simulink model "KIT_pr_UDR"  (R2023a)
settings: Solver=VariableStepAuto  StartTime=0.0  StopTime=inf  RelTol=1e-3
values from neighbouring files (symbols this model uses):
  Cx_alpha = [-0.0016 -0.0039 0.0346]    [KIT_UDR.mat]
  Cy_alpha = [-0.0006 0.0037 0.1555 0.2133]    [KIT_UDR.mat]
  InertiaTensor = [0.41697  0  0; 0  0.27367  0; 0  0  0.15697]    [KIT_UDR.mat]
  Mass = 3    [KIT_UDR.mat]
  mz_alpha = [-2e-05 0.0001 -0.0017 0.0042]    [KIT_UDR.mat]
  square = 0.228    [KIT_UDR.mat]
undefined symbols (not defined in the file or in its folder): deg, e0_0, e1_0, e2_0, e3_0, PitchAngleToTorque, rad, RollAngleToTorque, s, YawAngleToTorque
libraries: aerolibconvert2 x9, dsppolyfun x3, aerolibanimutils x3, sharedutil x2, etargetslib x1, aerolibutil x1, dspnetwork x1
settings Model: Creator=Sony  LastModifiedBy=sasha
settings SolverCC: AlgebraicLoopSolver=TrustRegion  DecoupledContinuousIntegration=on  MinimalZcImpactIntegration=on
settings DebuggingCC: ReadBeforeWriteMsg=DisableAll  WriteAfterWriteMsg=DisableAll  WriteAfterReadMsg=DisableAll  MultiTaskDSMMsg=none  UnconnectedInputMsg=warning  UnconnectedOutputMsg=warning  UnconnectedLineMsg=warning  ArithmeticOperatorsInVariantConditions=warning
settings ModelReferenceCC: UpdateModelReferenceTargets=IfOutOfDate  EnableRefExpFcnMdlSchedulingChecks=on
settings SFSimCC: SFSimEcho=off  CustomCodeUndefinedFunction=UseInterfaceOnly
settings RTWCC: DLArmComputeVersion=19.05
settings CodeAppCC: StateflowObjectComments=on

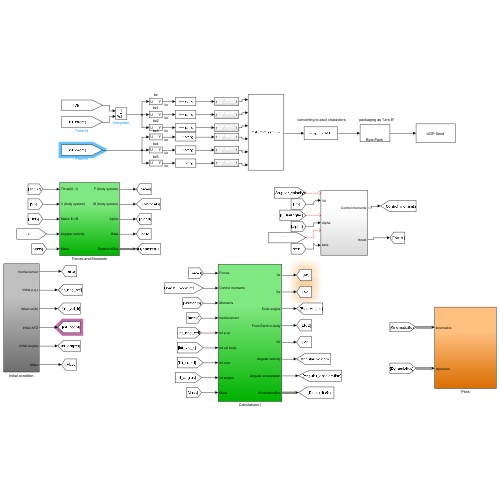
[thumbnail: Simulink's stored preview of the top-level diagram]
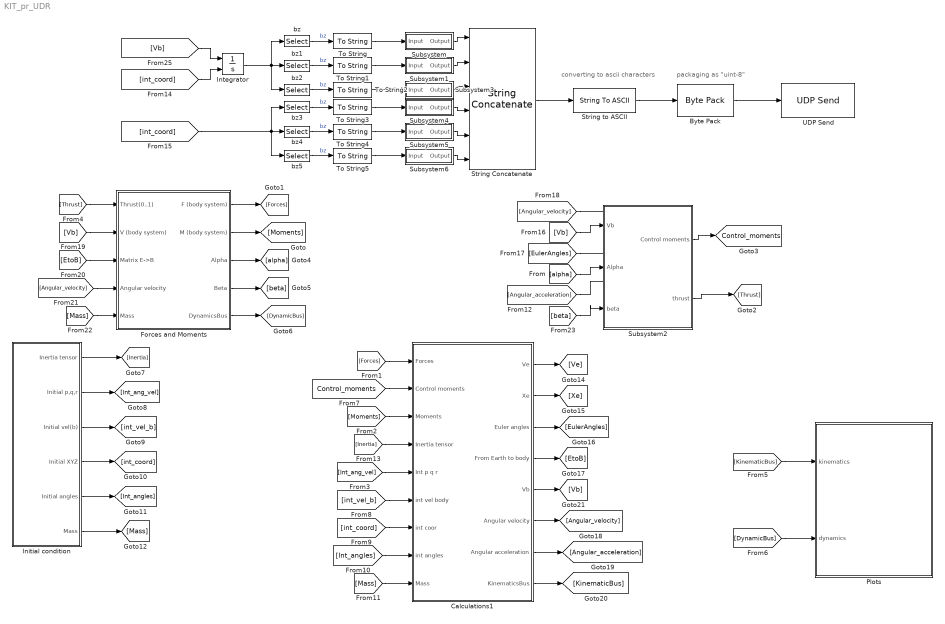
== system KIT_pr_UDR ==
  note: packaging as "uint-8"
  note: converting to ascii characters
  Byte Pack : etargetslib/Byte Pack  datatypes={'uint8'}  byteAlign=1
  Calculations1 : Subsystem
  Forces and Moments : Subsystem
  Initial condition : Subsystem
  Integrator : Integrator  InitialConditionSource=external
  Plots : Subsystem
  String Concatenate : StringConcatenate  Inputs=6
  String to ASCII : StringToASCII  OutputVectorSize=64
  Subsystem : Subsystem
  Subsystem1 : Subsystem
  Subsystem2 : Subsystem
  Subsystem3 : Subsystem
  Subsystem4 : Subsystem
  Subsystem5 : Subsystem
  Subsystem6 : Subsystem
  To String{,1..5} (6 alike) : ToString
  UDP Send : dspnetwork/UDP Send  remoteURL='127.0.0.1'  remotePort=1234  localURL='0.0.0.0'  localPortSource=Automatically determine  localPort=-1  sendBufferSize=8192  sampletime=-1  blockPlatform=[]  separateLengthPort=0
      settings: LibrarySourceBlock=dspsnks4/UDP Send
  bz : Selector  InputPortWidth=3  IndexOptions=Index vector (dialog)  Indices=1  OutputSizes=1
  bz1 : Selector  InputPortWidth=3  IndexOptions=Index vector (dialog)  Indices=2  OutputSizes=1
  bz2 : Selector  InputPortWidth=3  IndexOptions=Index vector (dialog)  Indices=3  OutputSizes=1
  bz3 : Selector  InputPortWidth=3  IndexOptions=Index vector (dialog)  Indices=1  OutputSizes=1
  bz4 : Selector  InputPortWidth=3  IndexOptions=Index vector (dialog)  Indices=2  OutputSizes=1
  bz5 : Selector  InputPortWidth=3  IndexOptions=Index vector (dialog)  Indices=3  OutputSizes=1
  tag scope: Control_moments=global
  wires:
  [Forces] -> Calculations1/1(Forces)
  Forces and Moments/1(F (body system)) -> [Forces]
  Subsystem2/1(Control moments) -> [Control_moments]
  Subsystem2/2(thrust) -> [Thrust]
  [Control_moments] -> Calculations1/2(Control moments)
  Forces and Moments/2(M (body system)) -> [Moments]
  Forces and Moments/3(Alpha) -> [alpha]
  Forces and Moments/4(Beta) -> [beta]
  Forces and Moments/5(DynamicsBus) -> [DynamicBus]
  [alpha] -> Subsystem2/2(Alpha)
  [DynamicBus] -> Plots/2(dynamics)
  [Moments] -> Calculations1/3(Moments)
  [Thrust] -> Forces and Moments/1(Thrust(0..1))
  Initial condition/1(Inertia tensor) -> [Inertia]
  Initial condition/2(Initial p,q,r) -> [Int_ang_vel]
  Initial condition/3(Initial vel(b)) -> [int_vel_b]
  Initial condition/4(Initial XYZ) -> [int_coord]
  Initial condition/5(Initial angles) -> [Int_angles]
  Initial condition/6(Mass) -> [Mass]
  Calculations1/1(Ve) -> [Ve]
  Calculations1/2(Xe) -> [Xe]
  Calculations1/3(Euler angles) -> [EulerAngles]
  Calculations1/4(From Earth to body) -> [EtoB]
  Calculations1/8(KinematicsBus) -> [KinematicBus]
  Calculations1/6(Angular velocity) -> [Angular_velocity]
  Calculations1/7(Angular acceleration) -> [Angular_acceleration]
  Calculations1/5(Vb) -> [Vb]
  [KinematicBus] -> Plots/1(kinematics)
  [Mass] -> Calculations1/9(Mass)
  [Int_angles] -> Calculations1/8(int angles)
  [int_coord] -> Calculations1/7("int coor ")
  [int_vel_b] -> Calculations1/6(int vel body)
  [Int_ang_vel] -> Calculations1/5(Int p q r)
  [Inertia] -> Calculations1/4(Inertia tensor)
  [EulerAngles] -> ?
  [Vb] -> Subsystem2/1(Vb)
  [Angular_velocity] -> ?
  [Vb] -> Forces and Moments/2(V (body system))
  [Mass] -> Forces and Moments/5(Mass)
  [Angular_velocity] -> Forces and Moments/4(Angular velocity)
  [EtoB] -> Forces and Moments/3(Matrix E->B)
  [Angular_acceleration] -> ?
  [beta] -> Subsystem2/3(beta)
  Subsystem3/1(Output) -> String Concatenate/3
  To String5/1 -> Subsystem6/1(Input)
  bz4/1 -> To String4/1  "bz"
  bz5/1 -> To String5/1  "bz"
  To String4/1 -> Subsystem5/1(Input)
  bz3/1 -> To String3/1  "bz"
  To String3/1 -> Subsystem4/1(Input)
  Subsystem1/1(Output) -> String Concatenate/2
  [int_coord] -> bz5/1, bz4/1, bz3/1
  Subsystem5/1(Output) -> String Concatenate/5
  bz1/1 -> To String1/1  "bz"
  Subsystem/1(Output) -> String Concatenate/1
  To String/1 -> Subsystem/1(Input)
  bz/1 -> To String/1  "bz"
  To String1/1 -> Subsystem1/1(Input)
  Subsystem6/1(Output) -> String Concatenate/6
  Byte Pack/1 -> UDP Send/1
  Integrator/1 -> bz2/1, bz/1, bz1/1
  Subsystem4/1(Output) -> String Concatenate/4
  bz2/1 -> To String2/1  "bz"
  String Concatenate/1 -> String to ASCII/1
  To String2/1 -> Subsystem3/1(Input)
  String to ASCII/1 -> Byte Pack/1
  [int_coord] -> Integrator/2
  [Vb] -> Integrator/1

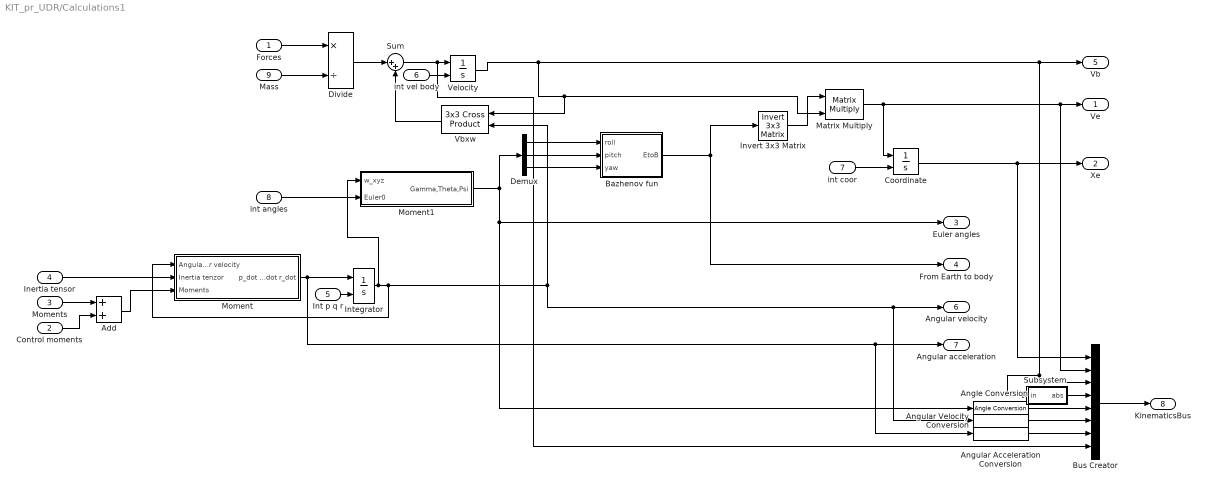
== system KIT_pr_UDR/Calculations1 ==
  Forces : Inport
  Control moments : Inport  Port=2
  Moments : Inport  Port=3
  Inertia tensor : Inport  Port=4
  Int p q r : Inport  Port=5
  int vel body : Inport  Port=6
  "int coor " : Inport  Port=7
  int angles : Inport  Port=8
  Mass : Inport  Port=9
  Add : Sum
  Angle Conversion : aerolibconvert2/Angle Conversion  IU=rad  OU=deg
  Angular Acceleration Conversion : aerolibconvert2/Angular Acceleration Conversion  IU=deg/s^2  OU=rad/s^2
  Angular Velocity Conversion : aerolibconvert2/Angular Velocity Conversion  IU=rad/s  OU=deg/s
  Bazhenov fun : MATLAB Function  TreatAsAtomicUnit=on
  Bus Creator : BusCreator  Inputs=8
  Coordinate : Integrator  InitialConditionSource=external
  Demux : Demux  Outputs=3
  Divide : Product  Inputs=*/
  Integrator : Integrator  InitialConditionSource=external
  Invert 3x3 Matrix : aerolibutil/Invert  3x3 Matrix
  Matrix Multiply : Product  Multiplication=Matrix(*)
  Moment : Subsystem
  Moment1 : Subsystem
  Subsystem : Subsystem
  Sum : Sum  Inputs=|++
  Vbxw : sharedutil/3x3 Cross Product  aMode=aMode
  Velocity : Integrator  InitialConditionSource=external
  Ve : Outport  VectorParamsAs1DForOutWhenUnconnected=off
  Xe : Outport  Port=2  VectorParamsAs1DForOutWhenUnconnected=off
  Euler angles : Outport  Port=3  VectorParamsAs1DForOutWhenUnconnected=off
  From Earth to body : Outport  Port=4  VectorParamsAs1DForOutWhenUnconnected=off
  Vb : Outport  Port=5  VectorParamsAs1DForOutWhenUnconnected=off
  Angular velocity : Outport  Port=6  VectorParamsAs1DForOutWhenUnconnected=off
  Angular acceleration : Outport  Port=7  VectorParamsAs1DForOutWhenUnconnected=off
  KinematicsBus : Outport  Port=8  VectorParamsAs1DForOutWhenUnconnected=off
  wires:
  Forces/1 -> Divide/1
  Divide/1 -> Sum/1
  Sum/1 -> Bus Creator/8, Velocity/1
  Invert 3x3 Matrix/1 -> Matrix Multiply/1
  Moment/1(p_dot q_dot r_dot) -> Integrator/1, Angular Acceleration Conversion/1, Angular acceleration/1
  Inertia tensor/1 -> Moment/2(Inertia tenzor)
  Velocity/1 -> Matrix Multiply/2, Vbxw/1, Subsystem/1(in), Bus Creator/3, Vb/1
  Integrator/1 -> Moment1/1(w_xyz), Moment/1(Angular velocity), Vbxw/2, Angular Velocity Conversion/1, Angular velocity/1
  Vbxw/1 -> Sum/2
  Int p q r/1 -> Integrator/2
  int vel body/1 -> Velocity/2
  "int coor "/1 -> Coordinate/2
  Moments/1 -> Add/1
  Control moments/1 -> Add/2
  Add/1 -> Moment/3(Moments)
  Bus Creator/1 -> KinematicsBus/1
  Coordinate/1 -> Bus Creator/1, Xe/1
  Matrix Multiply/1 -> Coordinate/1, Bus Creator/2, Ve/1
  Subsystem/1(abs) -> Bus Creator/4
  Angle Conversion/1 -> Bus Creator/5
  Angular Velocity Conversion/1 -> Bus Creator/6
  Angular Acceleration Conversion/1 -> Bus Creator/7
  Demux/2 -> Bazhenov fun/2(pitch)
  Demux/1 -> Bazhenov fun/1(roll)
  Demux/3 -> Bazhenov fun/3(yaw)
  Bazhenov fun/1(EtoB) -> From Earth to body/1, Invert 3x3 Matrix/1
  int angles/1 -> Moment1/2(Euler0)
  Moment1/1(Gamma,Theta,Psi) -> Angle Conversion/1, Euler angles/1, Demux/1
  Mass/1 -> Divide/2

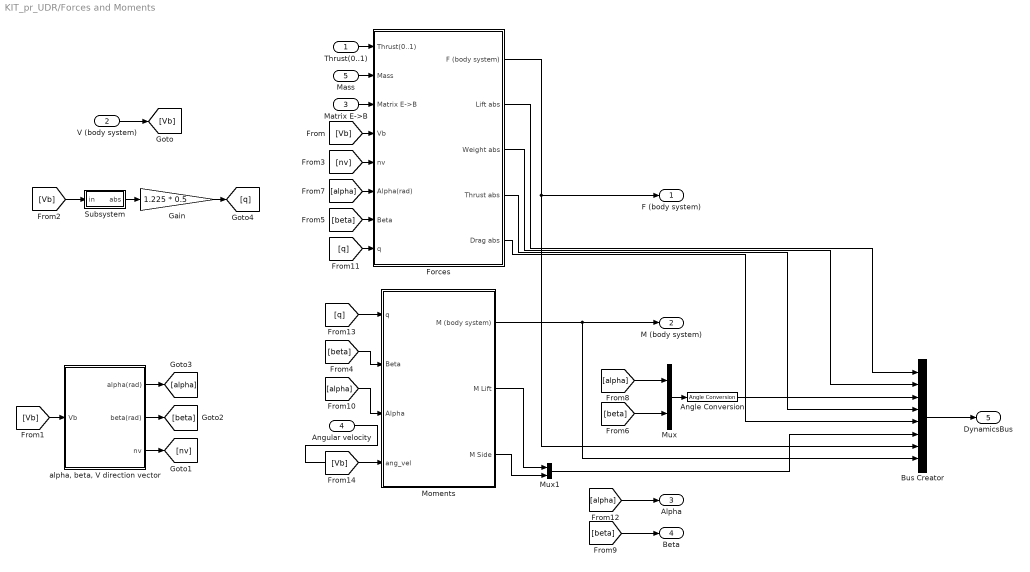
== system KIT_pr_UDR/Forces and Moments ==
  Thrust(0..1) : Inport
  V (body system) : Inport  Port=2
  Matrix E->B : Inport  Port=3
  Angular velocity : Inport  Port=4
  Mass : Inport  Port=5
  Angle Conversion : aerolibconvert2/Angle Conversion  IU=rad  OU=deg
  Bus Creator : BusCreator  Inputs=8
  Forces : Subsystem
  Gain : Gain  Gain=1.225 * 0.5
  Moments : Subsystem
  Mux : Mux  Inputs=2
  Mux1 : Mux  Inputs=2
  Subsystem : Subsystem
  "alpha, beta, V direction vector" : Subsystem
  F (body system) : Outport  VectorParamsAs1DForOutWhenUnconnected=off
  M (body system) : Outport  Port=2  VectorParamsAs1DForOutWhenUnconnected=off
  Alpha : Outport  Port=3  VectorParamsAs1DForOutWhenUnconnected=off
  Beta : Outport  Port=4  VectorParamsAs1DForOutWhenUnconnected=off
  DynamicsBus : Outport  Port=5  VectorParamsAs1DForOutWhenUnconnected=off
  wires:
  Thrust(0..1)/1 -> Forces/1(Thrust(0..1))
  Forces/1(F (body system)) -> F (body system)/1, Bus Creator/7
  Moments/1(M (body system)) -> Bus Creator/8, M (body system)/1
  V (body system)/1 -> [Vb]
  Matrix E->B/1 -> Forces/3(Matrix E->B)
  Bus Creator/1 -> DynamicsBus/1
  Forces/2(Lift abs) -> Bus Creator/1
  Forces/3(Weight abs) -> Bus Creator/2
  Mux/1 -> Angle Conversion/1
  Angle Conversion/1 -> Bus Creator/3
  Forces/4(Thrust abs) -> Bus Creator/4
  Forces/5(Drag abs) -> Bus Creator/5
  Mux1/1 -> Bus Creator/6
  Moments/2(M Lift) -> Mux1/1
  Moments/3(M Side) -> Mux1/2
  Mass/1 -> Forces/2(Mass)
  Gain/1 -> [q]
  Angular velocity/1 -> Moments/4(ang_vel)
  Subsystem/1(abs) -> Gain/1
  [Vb] -> Forces/4(Vb)
  [Vb] -> "alpha, beta, V direction vector"/1(Vb)
  [Vb] -> Subsystem/1(in)
  [nv] -> Forces/5(nv)
  "alpha, beta, V direction vector"/3(nv) -> [nv]
  "alpha, beta, V direction vector"/2(beta(rad)) -> [beta]
  [beta] -> Moments/2(Beta)
  [beta] -> Forces/7(Beta)
  [beta] -> Mux/2
  [beta] -> Beta/1
  "alpha, beta, V direction vector"/1(alpha(rad)) -> [alpha]
  [alpha] -> Forces/6(Alpha(rad))
  [alpha] -> Mux/1
  [alpha] -> Moments/3(Alpha)
  [alpha] -> Alpha/1
  [q] -> Forces/8(q)
  [q] -> Moments/1(q)
  [Vb] -> ?

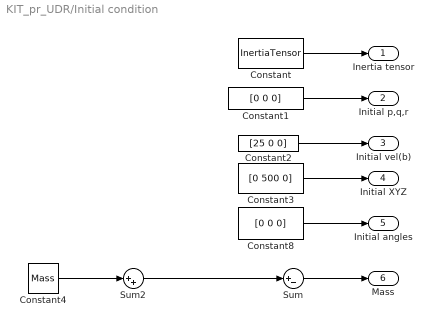
== system KIT_pr_UDR/Initial condition ==
  Constant : Constant  Value=InertiaTensor
  Constant1 : Constant  Value=[0 0 0]
  Constant2 : Constant  Value=[25 0 0]
  Constant3 : Constant  Value=[0 500 0]
  Constant4 : Constant  Value=Mass
  Constant8 : Constant  Value=[0 0 0]
  Sum : Sum  Inputs=|+-
  Sum2 : Sum  Inputs=|++
  Inertia tensor : Outport  VectorParamsAs1DForOutWhenUnconnected=off
  Initial p,q,r : Outport  Port=2  VectorParamsAs1DForOutWhenUnconnected=off
  Initial vel(b) : Outport  Port=3  VectorParamsAs1DForOutWhenUnconnected=off
  Initial XYZ : Outport  Port=4  VectorParamsAs1DForOutWhenUnconnected=off
  Initial angles : Outport  Port=5  VectorParamsAs1DForOutWhenUnconnected=off
  Mass : Outport  Port=6  VectorParamsAs1DForOutWhenUnconnected=off
  wires:
  Constant8/1 -> Initial angles/1
  Constant2/1 -> Initial vel(b)/1
  Constant3/1 -> Initial XYZ/1
  Constant1/1 -> Initial p,q,r/1
  Constant/1 -> Inertia tensor/1
  Sum/1 -> Mass/1
  Constant4/1 -> Sum2/1
  Sum2/1 -> Sum/1

== system KIT_pr_UDR/Plots ==
  kinematics : Inport
  dynamics : Inport  Port=2
  Bus Selector : BusSelector  OutputSignals=signal1,signal2,signal3,signal4,signal5,signal6,signal7,signal8
  Bus Selector1 : BusSelector  OutputSignals=signal1,signal2,signal3,signal4,signal5,signal6,signal7,signal8
  Dynamics : Scope  NumInputPorts=8
  Kinematics : Scope  NumInputPorts=8
  wires:
  kinematics/1 -> Bus Selector/1
  Bus Selector/1 -> Kinematics/1  "<signal1>"
  Bus Selector/2 -> Kinematics/2  "<signal2>"
  Bus Selector/3 -> Kinematics/3  "<signal3>"
  Bus Selector/4 -> Kinematics/4  "<signal4>"
  Bus Selector/5 -> Kinematics/5  "<signal5>"
  Bus Selector/6 -> Kinematics/6  "<signal6>"
  Bus Selector/7 -> Kinematics/7  "<signal7>"
  Bus Selector/8 -> Kinematics/8  "<signal8>"
  Bus Selector1/1 -> Dynamics/1  "<signal1>"
  Bus Selector1/2 -> Dynamics/2  "<signal2>"
  Bus Selector1/3 -> Dynamics/3  "<signal3>"
  Bus Selector1/4 -> Dynamics/4  "<signal4>"
  Bus Selector1/5 -> Dynamics/5  "<signal5>"
  Bus Selector1/6 -> Dynamics/6  "<signal6>"
  Bus Selector1/7 -> Dynamics/7  "<signal7>"
  Bus Selector1/8 -> Dynamics/8  "<signal8>"
  dynamics/1 -> Bus Selector1/1

== system KIT_pr_UDR/Subsystem ==
  Input : Inport
  String Concatenate1 : StringConcatenate
  String Constant : StringConstant  String="\",\""
  Output : Outport
  wires:
  Input/1 -> String Concatenate1/1
  String Constant/1 -> String Concatenate1/2
  String Concatenate1/1 -> Output/1

== system KIT_pr_UDR/Subsystem1 ==
  Input : Inport
  String Concatenate1 : StringConcatenate
  String Constant : StringConstant  String="\",\""
  Output : Outport
  wires:
  Input/1 -> String Concatenate1/1
  String Constant/1 -> String Concatenate1/2
  String Concatenate1/1 -> Output/1

== system KIT_pr_UDR/Subsystem2 ==
  Vb : Inport
  Alpha : Inport  Port=2
  beta : Inport  Port=3
  Angle Conversion : aerolibconvert2/Angle Conversion  IU=rad  OU=deg
  Angle Conversion1 : aerolibconvert2/Angle Conversion  IU=rad  OU=deg
  Constant : Constant  Value=25
  Stabilization+Autopilot : Subsystem  Commented=on
  Stabilization+Autopilot1 : Subsystem
  Thrust : Subsystem
  Control moments : Outport
  thrust : Outport  Port=2  VectorParamsAs1DForOutWhenUnconnected=off
  wires:
  Constant/1 -> Thrust/2(Target velocity)
  Stabilization+Autopilot1/1(Control Moment) -> Control moments/1
  Thrust/1(Thrust) -> thrust/1
  Vb/1 -> Thrust/1(Vb), Stabilization+Autopilot1/1(Vb)
  Alpha/1 -> Angle Conversion/1
  Angle Conversion/1 -> Stabilization+Autopilot1/2(alpha)
  beta/1 -> Angle Conversion1/1
  Angle Conversion1/1 -> Stabilization+Autopilot1/3(beta)

== system KIT_pr_UDR/Subsystem3 ==
  Input : Inport
  String Concatenate1 : StringConcatenate
  String Constant : StringConstant  String="\",\""
  Output : Outport
  wires:
  Input/1 -> String Concatenate1/1
  String Constant/1 -> String Concatenate1/2
  String Concatenate1/1 -> Output/1

== system KIT_pr_UDR/Subsystem4 ==
  Input : Inport
  String Concatenate1 : StringConcatenate
  String Constant : StringConstant  String="\",\""
  Output : Outport
  wires:
  Input/1 -> String Concatenate1/1
  String Constant/1 -> String Concatenate1/2
  String Concatenate1/1 -> Output/1

== system KIT_pr_UDR/Subsystem5 ==
  Input : Inport
  String Concatenate1 : StringConcatenate
  String Constant : StringConstant  String="\",\""
  Output : Outport
  wires:
  Input/1 -> String Concatenate1/1
  String Constant/1 -> String Concatenate1/2
  String Concatenate1/1 -> Output/1

== system KIT_pr_UDR/Subsystem6 ==
  Input : Inport
  String Concatenate1 : StringConcatenate
  String Constant : StringConstant  String="\",\""
  Output : Outport
  wires:
  Input/1 -> String Concatenate1/1
  String Constant/1 -> String Concatenate1/2
  String Concatenate1/1 -> Output/1

== system KIT_pr_UDR/Calculations1/Moment ==
  note: проверить транспонирование
  Angular velocity : Inport
  Inertia tenzor : Inport  Port=2
  Moments : Inport  Port=3
  3x3 Cross Product : sharedutil/3x3 Cross Product  aMode=aMode
  Matrix Divide : Product  Inputs=*/  Multiplication=Matrix(*)
  Matrix Multiply1 : Product  Multiplication=Matrix(*)
  Sum : Sum  Inputs=|-+
  Transpose : Math  Operator=transpose
  p_dot q_dot r_dot : Outport  VectorParamsAs1DForOutWhenUnconnected=off
  wires:
  Moments/1 -> Sum/2
  3x3 Cross Product/1 -> Sum/1
  Angular velocity/1 -> 3x3 Cross Product/1, Transpose/1
  Inertia tenzor/1 -> Matrix Multiply1/1, Matrix Divide/2
  Sum/1 -> Matrix Divide/1
  Matrix Divide/1 -> p_dot q_dot r_dot/1
  Matrix Multiply1/1 -> 3x3 Cross Product/2
  Transpose/1 -> Matrix Multiply1/2

== system KIT_pr_UDR/Calculations1/Moment1 ==
  w_xyz : Inport
  Euler0 : Inport  Port=2
  Selector : Selector  InputPortWidth=3  IndexOptions=Index vector (dialog)  Indices=[3 2 1]  OutputSizes=1
  Subsystem : Subsystem
  q0 q1 q2 q3 : Integrator  InitialConditionSource=external  InitialCondition=[e0_0 e1_0 e2_0 e3_0]
  q_dot : Subsystem
  Вычисление МНК : Subsystem  mask(Вычисление МНК){}
      mask help:
      | Вычисление направляющих косинусов из параметров кватерниона.
      | Блок рассчитан на использование российских обозначений и систем координат.
  Нормировка : Subsystem
  Переход к угловым координатам виртуальной реальности3 : Subsystem  mask(Вычисление кватерниона из углов Эйлера){}
      mask help:
      | Блок вычисления параметров кватерниона из углов Эйлера (рыскание, тангаж, крен в градусах).
      | Блок рассчитан на использование российских обозначений и систем координат.
      mask Display:
      | port_label('input',1,'\psi \vartheta \gamma [\circ]','Texmode','on')
      | port_label('output',1,'Q','Texmode','on')
  Gamma,Theta,Psi : Outport
  wires:
  q0 q1 q2 q3/1 -> Нормировка/1(Q)
  q_dot/1(qdot) -> q0 q1 q2 q3/1
  Вычисление МНК/1(МНК) -> Subsystem/1(МНК)
  Subsystem/1(Gama Theta Psi) -> Gamma,Theta,Psi/1
  w_xyz/1 -> q_dot/1(wx wy wz)
  Selector/1 -> Переход к угловым координатам виртуальной реальности3/1("Psi, Theta, Gamma")
  Переход к угловым координатам виртуальной реальности3/1(Q) -> q0 q1 q2 q3/2
  Euler0/1 -> Selector/1
  Нормировка/1(Qnorm) -> Вычисление МНК/1(Кват. Q), q_dot/2(q0 q1 q2 q3)

== system KIT_pr_UDR/Calculations1/Subsystem ==
  in : Inport
  Sqrt1 : Sqrt
  Square : Math  Operator=square
  Sum of Elements : Sum  Inputs=+
  abs : Outport  VectorParamsAs1DForOutWhenUnconnected=off
  wires:
  in/1 -> Square/1
  Square/1 -> Sum of Elements/1
  Sum of Elements/1 -> Sqrt1/1
  Sqrt1/1 -> abs/1

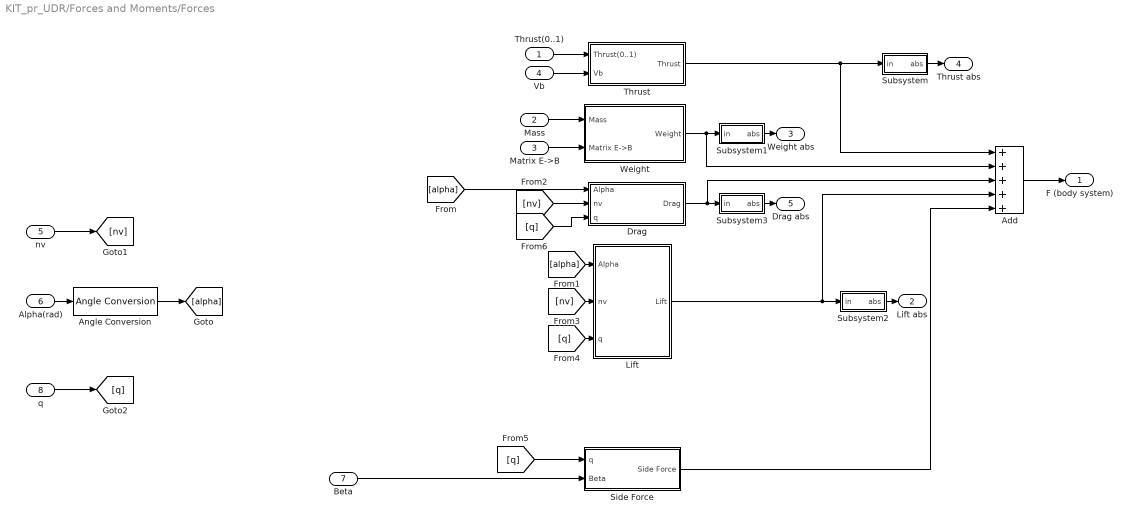
== system KIT_pr_UDR/Forces and Moments/Forces ==
  Thrust(0..1) : Inport
  Mass : Inport  Port=2
  Matrix E->B : Inport  Port=3
  Vb : Inport  Port=4
  nv : Inport  Port=5
  Alpha(rad) : Inport  Port=6
  Beta : Inport  Port=7
  q : Inport  Port=8
  Add : Sum  Inputs=5
  Angle Conversion : aerolibconvert2/Angle Conversion  IU=rad  OU=deg
  Drag : Subsystem
  Lift : Subsystem
  Side Force : Subsystem
  Subsystem : Subsystem
  Subsystem1 : Subsystem
  Subsystem2 : Subsystem
  Subsystem3 : Subsystem
  Thrust : Subsystem
  Weight : Subsystem
  F (body system) : Outport  VectorParamsAs1DForOutWhenUnconnected=off
  Lift abs : Outport  Port=2  VectorParamsAs1DForOutWhenUnconnected=off
  Weight abs : Outport  Port=3  VectorParamsAs1DForOutWhenUnconnected=off
  Thrust abs : Outport  Port=4  VectorParamsAs1DForOutWhenUnconnected=off
  Drag abs : Outport  Port=5  VectorParamsAs1DForOutWhenUnconnected=off
  wires:
  Add/1 -> F (body system)/1
  Weight/1(Weight) -> Subsystem1/1(in), Add/2
  Drag/1(Drag) -> Add/3, Subsystem3/1(in)
  Lift/1(Lift) -> Subsystem2/1(in), Add/4
  Vb/1 -> Thrust/2(Vb)
  nv/1 -> [nv]
  Alpha(rad)/1 -> Angle Conversion/1
  Mass/1 -> Weight/1(Mass)
  Matrix E->B/1 -> Weight/2(Matrix E->B)
  Thrust(0..1)/1 -> Thrust/1(Thrust(0..1))
  Subsystem1/1(abs) -> Weight abs/1
  Subsystem2/1(abs) -> Lift abs/1
  Subsystem/1(abs) -> Thrust abs/1
  Subsystem3/1(abs) -> Drag abs/1
  Thrust/1(Thrust) -> Subsystem/1(in), Add/1
  Beta/1 -> Side Force/2(Beta)
  Angle Conversion/1 -> [alpha]
  Side Force/1(Side Force) -> Add/5
  [alpha] -> Drag/1(Alpha)
  [alpha] -> Lift/1(Alpha)
  [nv] -> Drag/2(nv)
  [nv] -> Lift/2(nv)
  q/1 -> [q]
  [q] -> Lift/3(q)
  [q] -> Drag/3(q)
  [q] -> Side Force/1(q)

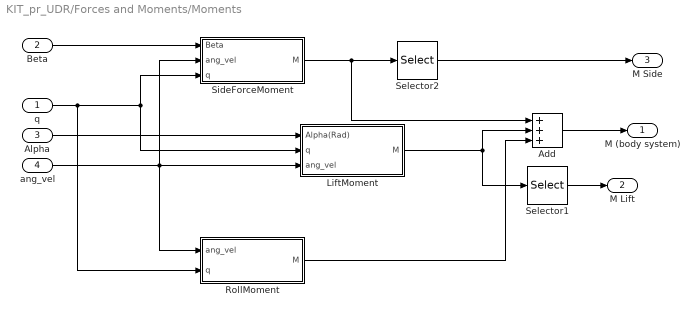
== system KIT_pr_UDR/Forces and Moments/Moments ==
  q : Inport
  Beta : Inport  Port=2
  Alpha : Inport  Port=3
  ang_vel : Inport  Port=4
  Add : Sum  Inputs=+++
  LiftMoment : Subsystem
  RollMoment : Subsystem
  Selector1 : Selector  InputPortWidth=3  IndexOptions=Index vector (dialog)  Indices=3  OutputSizes=1
  Selector2 : Selector  InputPortWidth=3  IndexOptions=Index vector (dialog)  Indices=2  OutputSizes=1
  SideForceMoment : Subsystem
  M (body system) : Outport  VectorParamsAs1DForOutWhenUnconnected=off
  M Lift : Outport  Port=2  VectorParamsAs1DForOutWhenUnconnected=off
  M Side : Outport  Port=3  VectorParamsAs1DForOutWhenUnconnected=off
  wires:
  Add/1 -> M (body system)/1
  LiftMoment/1(M) -> Add/2, Selector1/1
  q/1 -> RollMoment/2(q), SideForceMoment/3(q), LiftMoment/2(q)
  Alpha/1 -> LiftMoment/1(Alpha(Rad))
  Beta/1 -> SideForceMoment/1(Beta)
  Selector1/1 -> M Lift/1
  Selector2/1 -> M Side/1
  ang_vel/1 -> SideForceMoment/2(ang_vel), LiftMoment/3(ang_vel), RollMoment/1(ang_vel)
  RollMoment/1(M) -> Add/3
  SideForceMoment/1(M) -> Add/1, Selector2/1

== system KIT_pr_UDR/Forces and Moments/Subsystem ==
  in : Inport
  Square : Math  Operator=square
  Sum of Elements : Sum  Inputs=+
  abs : Outport  VectorParamsAs1DForOutWhenUnconnected=off
  wires:
  in/1 -> Square/1
  Square/1 -> Sum of Elements/1
  Sum of Elements/1 -> abs/1

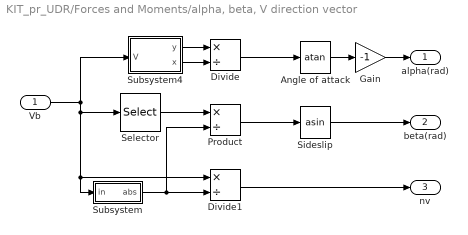
== system KIT_pr_UDR/Forces and Moments/alpha, beta, V direction vector ==
  Vb : Inport
  Angle of attack : Trigonometry  Operator=atan
  Divide : Product  Inputs=*/
  Divide1 : Product  Inputs=*/
  Gain : Gain  Gain=-1
  Product : Product  Inputs=*/  SaturateOnIntegerOverflow=on  OutDataTypeStr=Inherit: Same as first input
  Selector : Selector  InputPortWidth=3  IndexOptions=Index vector (dialog)  Indices=[3]  OutputSizes=1
  Sideslip : Trigonometry  Operator=asin  OutputSignalType=real
  Subsystem : Subsystem
  Subsystem4 : Subsystem
  alpha(rad) : Outport  VectorParamsAs1DForOutWhenUnconnected=off
  beta(rad) : Outport  Port=2  VectorParamsAs1DForOutWhenUnconnected=off
  nv : Outport  Port=3  VectorParamsAs1DForOutWhenUnconnected=off
  wires:
  Divide/1 -> Angle of attack/1
  Subsystem4/1(y) -> Divide/1
  Selector/1 -> Product/1
  Subsystem4/2(x) -> Divide/2
  Divide1/1 -> nv/1
  Product/1 -> Sideslip/1
  Angle of attack/1 -> Gain/1
  Subsystem/1(abs) -> Product/2, Divide1/2
  Vb/1 -> Selector/1, Subsystem/1(in), Divide1/1, Subsystem4/1(V)
  Gain/1 -> alpha(rad)/1
  Sideslip/1 -> beta(rad)/1

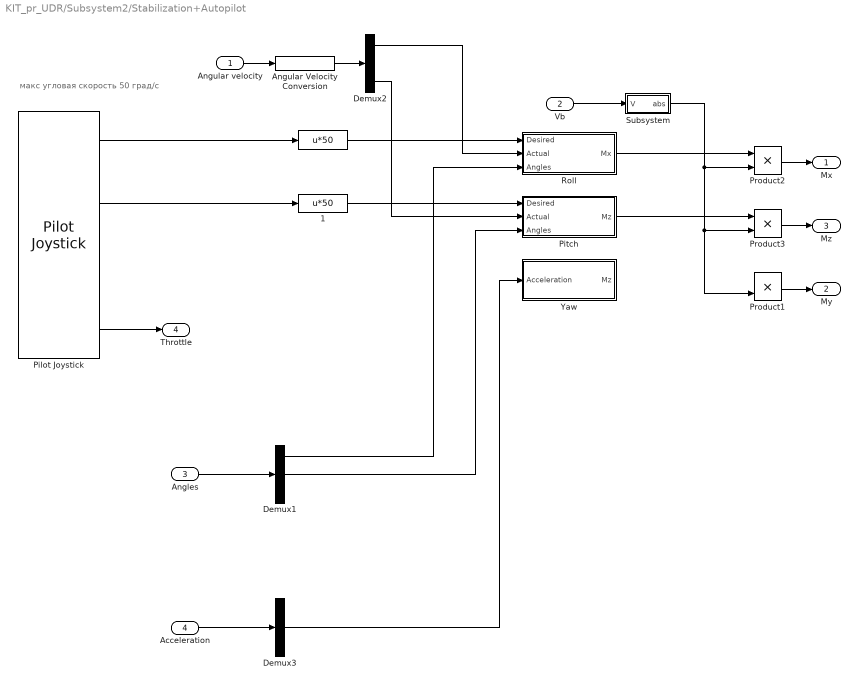
== system KIT_pr_UDR/Subsystem2/Stabilization+Autopilot ==
  note: макс угловая скорость 50 град/с
  Angular velocity : Inport
  Vb : Inport  Port=2
  Angles : Inport  Port=3
  Acceleration : Inport  Port=4
  " " : Fcn  Expr=u*50
  " 1" : Fcn  Expr=u*50
  Angular Velocity Conversion : aerolibconvert2/Angular Velocity Conversion  IU=rad/s  OU=deg/s
  Demux1 : Demux  Outputs=3
  Demux2 : Demux  Outputs=3
  Demux3 : Demux  Outputs=3
  Pilot Joystick : aerolibanimutils/Pilot Joystick  JoystickID=Joystick1  OutputConfiguration=FourAxis  SampleTime=1/30
  Pitch : Subsystem
  Product1 : Product
  Product2 : Product
  Product3 : Product
  Roll : Subsystem
  Subsystem : Subsystem
  Yaw : Subsystem
  Mx : Outport
  My : Outport  Port=2
  Mz : Outport  Port=3
  Throttle : Outport  Port=4
  wires:
  Subsystem/1(abs) -> Product1/2, Product3/2, Product2/2
  Vb/1 -> Subsystem/1(V)
  Product2/1 -> Mx/1
  " 1"/1 -> Pitch/1(Desired)
  Demux2/3 -> Pitch/2(Actual)
  Angular Velocity Conversion/1 -> Demux2/1
  Demux2/1 -> Roll/2(Actual)
  " "/1 -> Roll/1(Desired)
  Product1/1 -> My/1
  Angular velocity/1 -> Angular Velocity Conversion/1
  Pilot Joystick/1 -> " "/1
  Pilot Joystick/2 -> " 1"/1
  Angles/1 -> Demux1/1
  Demux1/1 -> Roll/3(Angles)
  Demux1/2 -> Pitch/3(Angles)
  Pitch/1(Mz) -> Product3/1
  Roll/1(Mx) -> Product2/1
  Acceleration/1 -> Demux3/1
  Demux3/2 -> Yaw/1(Acceleration)
  Pilot Joystick/4 -> Throttle/1
  Product3/1 -> Mz/1

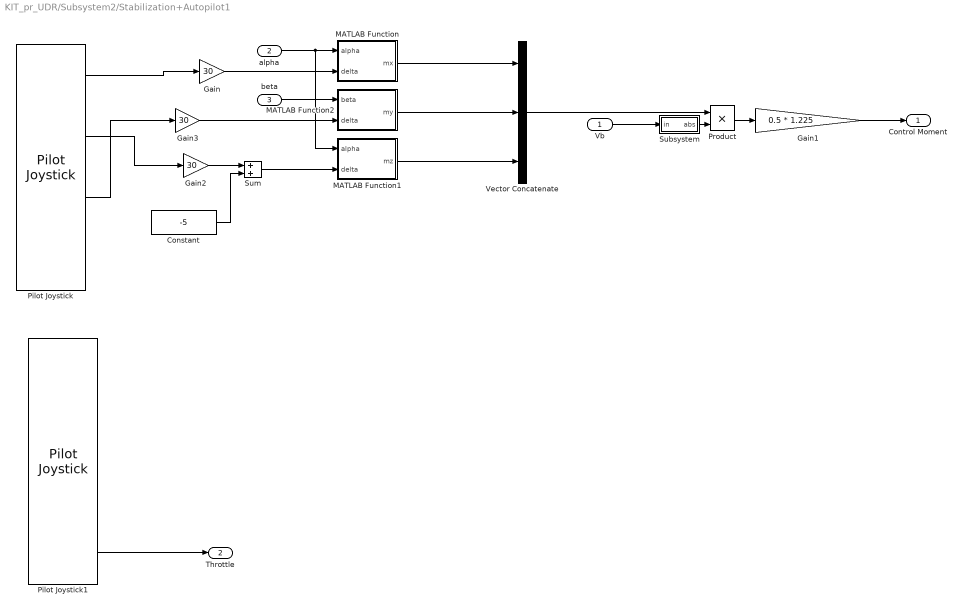
== system KIT_pr_UDR/Subsystem2/Stabilization+Autopilot1 ==
  Vb : Inport
  alpha : Inport  Port=2
  beta : Inport  Port=3
  Constant : Constant  Value=-5
  Gain : Gain  Gain=30
  Gain1 : Gain  Gain=0.5 * 1.225
  Gain2 : Gain  Gain=30
  Gain3 : Gain  Gain=30
  MATLAB Function : MATLAB Function  TreatAsAtomicUnit=on
  MATLAB Function1 : MATLAB Function  TreatAsAtomicUnit=on
  MATLAB Function2 : MATLAB Function  TreatAsAtomicUnit=on
  Pilot Joystick : aerolibanimutils/Pilot Joystick  JoystickID=Joystick1  OutputConfiguration=FourAxis  SampleTime=1/30
  Pilot Joystick1 : aerolibanimutils/Pilot Joystick  JoystickID=Joystick2  OutputConfiguration=FourAxis  SampleTime=1/30
  Product : Product
  Subsystem : Subsystem
  Sum : Sum
  Vector Concatenate : Concatenate  NumInputs=3
  Control Moment : Outport
  Throttle : Outport  Port=2
  wires:
  Vb/1 -> Subsystem/1(in)
  Gain/1 -> MATLAB Function/2(delta)
  alpha/1 -> MATLAB Function1/1(alpha), MATLAB Function/1(alpha)
  MATLAB Function/1(mx) -> Vector Concatenate/1
  Vector Concatenate/1 -> Product/1
  Subsystem/1(abs) -> Product/2
  Product/1 -> Gain1/1
  Constant/1 -> Sum/2
  MATLAB Function1/1(mz) -> Vector Concatenate/3
  Sum/1 -> MATLAB Function1/2(delta)
  Gain2/1 -> Sum/1
  Gain1/1 -> Control Moment/1
  Pilot Joystick/2 -> Gain2/1
  Pilot Joystick/1 -> Gain/1
  beta/1 -> MATLAB Function2/1(beta)
  MATLAB Function2/1(my) -> Vector Concatenate/2
  Pilot Joystick/3 -> Gain3/1
  Gain3/1 -> MATLAB Function2/2(delta)
  Pilot Joystick1/4 -> Throttle/1

== system KIT_pr_UDR/Subsystem2/Thrust ==
  Vb : Inport
  Target velocity : Inport  Port=2
  Thrust control : Inport  Port=3
  Constant : Constant
  Constant1 : Constant  Value=-10
  Constant2 : Constant
  MATLAB Function : MATLAB Function  TreatAsAtomicUnit=on
  Subsystem : Subsystem
  Subtract : Sum  Inputs=+-
  Switch : Switch  Criteria=u2 > Threshold  SaturateOnIntegerOverflow=off  InputSameDT=off
  Thrust : Outport  VectorParamsAs1DForOutWhenUnconnected=off
  wires:
  MATLAB Function/1(y) -> Switch/1
  Subtract/1 -> MATLAB Function/1(x)
  Target velocity/1 -> Subtract/2
  Constant1/1 -> MATLAB Function/2(argument)
  Constant/1 -> MATLAB Function/3(amplitude)
  Thrust control/1 -> Switch/3
  Switch/1 -> Thrust/1
  Constant2/1 -> Switch/2
  Subsystem/1(abs) -> Subtract/1
  Vb/1 -> Subsystem/1(in)

== system KIT_pr_UDR/Calculations1/Moment1/Subsystem ==
  МНК : Inport
  Mux1 : Mux  Inputs=3
  Trigonometric Function : Trigonometry  Operator=asin
  Trigonometric Function1 : Trigonometry  Operator=atan2
  Trigonometric Function2 : Trigonometry  Operator=atan2
  ax (1) : Selector  InputPortWidth=9  IndexOptions=Index vector (dialog)  Indices=1  OutputSizes=1
  bx (4) : Selector  InputPortWidth=9  IndexOptions=Index vector (dialog)  Indices=4  OutputSizes=1
  by (5) : Selector  InputPortWidth=9  IndexOptions=Index vector (dialog)  Indices=5  OutputSizes=1
  bz (6) : Selector  InputPortWidth=9  IndexOptions=Index vector (dialog)  Indices=6  OutputSizes=1
  dx (7) : Selector  InputPortWidth=9  IndexOptions=Index vector (dialog)  Indices=7  OutputSizes=1
  g : Gain  Gain=-1
  g1 : Gain
  Gama Theta Psi : Outport
  wires:
  Mux1/1 -> Gama Theta Psi/1
  Trigonometric Function/1 -> Mux1/2  "Theta"
  bx (4)/1 -> Trigonometric Function/1  "bx"
  g1/1 -> Mux1/3  "Psi"
  МНК/1 -> ax (1)/1, dx (7)/1, by (5)/1, bz (6)/1, bx (4)/1
  ax (1)/1 -> Trigonometric Function2/2
  Trigonometric Function2/1 -> g1/1
  dx (7)/1 -> Trigonometric Function2/1
  g/1 -> Mux1/1  "Gamma"
  bz (6)/1 -> Trigonometric Function1/1  "bz"
  by (5)/1 -> Trigonometric Function1/2  "by"
  Trigonometric Function1/1 -> g/1

== system KIT_pr_UDR/Calculations1/Moment1/q_dot ==
  note: dq0/dt  =  – (q1*wx  + q2*wy  +  q3*wz)/2
      | dq1/dt  =    (q0*wx  + q2*wz  –  q3*wy)/2
      | dq2/dt  =    (q0*wy  – q1*wz  +  q3*wx)/2
      | dq3/dt  =    (q0*wz  + q1*wy  –  q2*wx)/2
  note: u1 = wx
      | u2 = wy
      | u3 = wz
      | u4 = q0
      | u5 = q1
      | u6 = q2
      | u7 = q3
  wx wy wz : Inport
  q0 q1 q2 q3 : Inport  Port=2
  Mux1 : Mux  Inputs=[3 4]
  Mux2 : Mux
  q0dot = – (q1*wx  + q2*wy  +  q3*wz)/2 : Fcn  Expr=-0.5 * ( u[5]*u[1]+u[6]*u[2]+u[7]*u[3] )
  q1dot = (q0*wx  + q2*wz  –  q3*wy)/2 : Fcn  Expr=0.5 * ( u[4]*u[1]+u[6]*u[3]-u[7]*u[2] )
  q2dot = (q0*wy  – q1*wz  +  q3*wx)/2 : Fcn  Expr=0.5 * ( u[4]*u[2]+u[7]*u[1]-u[5]*u[3] )
  q3dot = (q0*wz  + q1*wy  –  q2*wx)/2 : Fcn  Expr=0.5 * ( u[4]*u[3]+u[5]*u[2]-u[6]*u[1] )
  qdot : Outport  InitialOutput=0
  wires:
  wx wy wz/1 -> Mux1/1
  Mux2/1 -> qdot/1
  q0dot = – (q1*wx  + q2*wy  +  q3*wz)/2/1 -> Mux2/1
  q1dot = (q0*wx  + q2*wz  –  q3*wy)/2/1 -> Mux2/2
  q2dot = (q0*wy  – q1*wz  +  q3*wx)/2/1 -> Mux2/3
  Mux1/1 -> q2dot = (q0*wy  – q1*wz  +  q3*wx)/2/1, q3dot = (q0*wz  + q1*wy  –  q2*wx)/2/1, q0dot = – (q1*wx  + q2*wy  +  q3*wz)/2/1, q1dot = (q0*wx  + q2*wz  –  q3*wy)/2/1
  q3dot = (q0*wz  + q1*wy  –  q2*wx)/2/1 -> Mux2/4
  q0 q1 q2 q3/1 -> Mux1/2

== system KIT_pr_UDR/Calculations1/Moment1/Вычисление МНК ==
  Кват. Q : Inport
  " Az = 2*(q1*q3 + q0*q2)" : Fcn  Expr=2*( u(2)*u(4)+u(1)*u(3) )
  Ax = q0*q0 + q1*q1 - q2*q2 - q3*q3 : Fcn  Expr=u(1)*u(1)+u(2)*u(2)-u(3)*u(3)-u(4)*u(4)
  Ay = 2*(q1*q2 - q0*q3) : Fcn  Expr=2*( u(2)*u(3)-u(1)*u(4) )
  Bx = 2*(q1*q2 + q0*q3) : Fcn  Expr=2*( u(2)*u(3)+u(1)*u(4) )
  By = q0*q0 - q1*q1 + q2*q2 - q3*q3 : Fcn  Expr=u(1)*u(1)-u(2)*u(2)+u(3)*u(3)-u(4)*u(4)
  Bz = 2*(q2*q3 - q0*q1) : Fcn  Expr=2*( u(3)*u(4)-u(1)*u(2) )
  Dx = 2*(q1*q3 - q0*q2) : Fcn  Expr=2*( u(2)*u(4)-u(1)*u(3) )
  Dy = 2*(q2*q3 + q0*q1) : Fcn  Expr=2*( u(3)*u(4)+u(1)*u(2) )
  Dz = q0*q0 - q1*q1 - q2*q2 + q3*q3 : Fcn  Expr=u(1)*u(1)-u(2)*u(2)-u(3)*u(3)+u(4)*u(4)
  Mux2 : Mux  Inputs=9
  МНК : Outport
  wires:
  Ax = q0*q0 + q1*q1 - q2*q2 - q3*q3/1 -> Mux2/1
  Ay = 2*(q1*q2 - q0*q3)/1 -> Mux2/2
  " Az = 2*(q1*q3 + q0*q2)"/1 -> Mux2/3
  Bx = 2*(q1*q2 + q0*q3)/1 -> Mux2/4
  By = q0*q0 - q1*q1 + q2*q2 - q3*q3/1 -> Mux2/5
  Bz = 2*(q2*q3 - q0*q1)/1 -> Mux2/6
  Dz = q0*q0 - q1*q1 - q2*q2 + q3*q3/1 -> Mux2/9
  Dx = 2*(q1*q3 - q0*q2)/1 -> Mux2/7
  Dy = 2*(q2*q3 + q0*q1)/1 -> Mux2/8
  Кват. Q/1 -> By = q0*q0 - q1*q1 + q2*q2 - q3*q3/1, Ax = q0*q0 + q1*q1 - q2*q2 - q3*q3/1, Ay = 2*(q1*q2 - q0*q3)/1, " Az = 2*(q1*q3 + q0*q2)"/1, Bx = 2*(q1*q2 + q0*q3)/1, Bz = 2*(q2*q3 - q0*q1)/1, Dx = 2*(q1*q3 - q0*q2)/1, Dz = q0*q0 - q1*q1 - q2*q2 + q3*q3/1, Dy = 2*(q2*q3 + q0*q1)/1
  Mux2/1 -> МНК/1

== system KIT_pr_UDR/Calculations1/Moment1/Нормировка ==
  Q : Inport
  Dot Product : DotProduct  OutDataTypeStr=Inherit: Inherit via internal rule
  Sqrt : Sqrt
  Нормировка : Product  Inputs=*/
  Qnorm : Outport
  wires:
  Q/1 -> Dot Product/1, Dot Product/2, Нормировка/1
  Dot Product/1 -> Sqrt/1
  Sqrt/1 -> Нормировка/2
  Нормировка/1 -> Qnorm/1

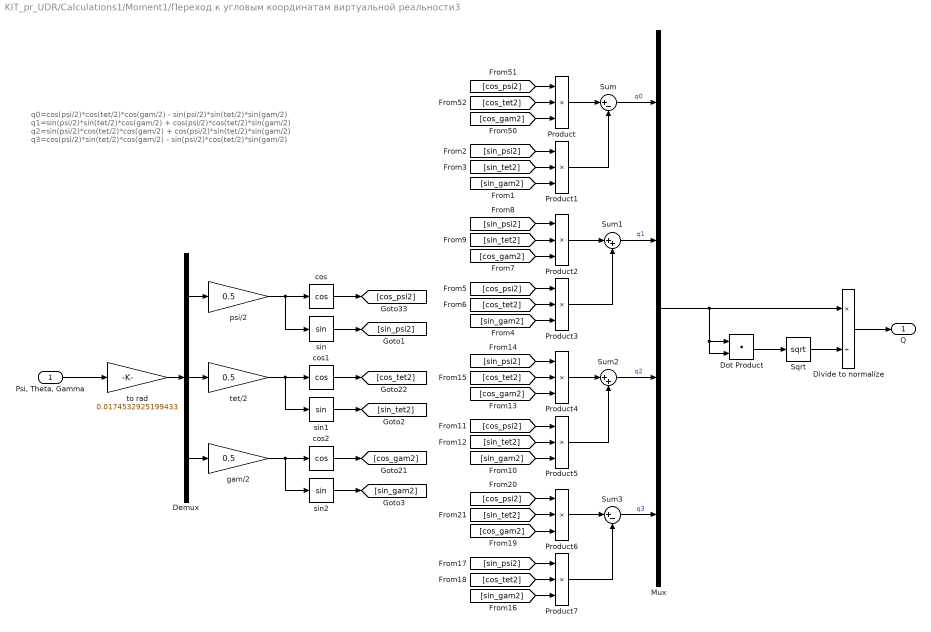
== system KIT_pr_UDR/Calculations1/Moment1/Переход к угловым координатам виртуальной реальности3 ==
  note: q0=cos(psi/2)*cos(tet/2)*cos(gam/2) - sin(psi/2)*sin(tet/2)*sin(gam/2)
      |     q1=sin(psi/2)*sin(tet/2)*cos(gam/2) + cos(psi/2)*cos(tet/2)*sin(gam/2)
      |     q2=sin(psi/2)*cos(tet/2)*cos(gam/2) + cos(psi/2)*sin(tet/2)*sin(gam/2)
      |     q3=cos(psi/2)*sin(tet/2)*cos(gam/2) - sin(psi/2)*cos(tet/2)*sin(gam/2)
  "Psi, Theta, Gamma" : Inport
  Demux : Demux  Outputs=3
  Divide to normalize : Product  Inputs=*/
  Dot Product : DotProduct  OutDataTypeStr=Inherit: Inherit via internal rule
  Mux : Mux
  Product{,1..7} (8 alike) : Product  Inputs=3  RndMeth=Zero
  Sqrt : Sqrt
  Sum : Sum  Inputs=|+-
  Sum1 : Sum  Inputs=|++
  Sum2 : Sum  Inputs=|++
  Sum3 : Sum  Inputs=|+-
  cos : Trigonometry  Operator=cos
  cos1 : Trigonometry  Operator=cos
  cos2 : Trigonometry  Operator=cos
  gam/2 : Gain  Gain=0.5
  psi/2 : Gain  Gain=0.5
  sin : Trigonometry
  sin1 : Trigonometry
  sin2 : Trigonometry
  tet/2 : Gain  Gain=0.5
  to rad : Gain  Gain=0.0174532925199433
  Q : Outport
  wires:
  cos/1 -> [cos_psi2]
  [cos_psi2] -> Product/1
  [cos_tet2] -> Product/2
  cos1/1 -> [cos_tet2]
  cos2/1 -> [cos_gam2]
  "Psi, Theta, Gamma"/1 -> to rad/1
  Demux/1 -> psi/2/1
  sin/1 -> [sin_psi2]
  Demux/2 -> tet/2/1
  sin1/1 -> [sin_tet2]
  Demux/3 -> gam/2/1
  sin2/1 -> [sin_gam2]
  to rad/1 -> Demux/1
  [cos_gam2] -> Product/3
  [sin_psi2] -> Product1/1
  [sin_tet2] -> Product1/2
  [sin_gam2] -> Product1/3
  Product/1 -> Sum/1
  Product1/1 -> Sum/2
  Sum/1 -> Mux/1  "q0"
  Mux/1 -> Dot Product/1, Dot Product/2, Divide to normalize/1
  [sin_psi2] -> Product2/1
  [sin_tet2] -> Product2/2
  [cos_gam2] -> Product2/3
  [cos_psi2] -> Product3/1
  [cos_tet2] -> Product3/2
  [sin_gam2] -> Product3/3
  Product2/1 -> Sum1/1
  Product3/1 -> Sum1/2
  Sum1/1 -> Mux/2  "q1"
  [sin_psi2] -> Product4/1
  [cos_tet2] -> Product4/2
  [cos_gam2] -> Product4/3
  [cos_psi2] -> Product5/1
  [sin_tet2] -> Product5/2
  [sin_gam2] -> Product5/3
  Product4/1 -> Sum2/1
  Product5/1 -> Sum2/2
  Sum2/1 -> Mux/3  "q2"
  [cos_psi2] -> Product6/1
  [sin_tet2] -> Product6/2
  [cos_gam2] -> Product6/3
  [sin_psi2] -> Product7/1
  [cos_tet2] -> Product7/2
  [sin_gam2] -> Product7/3
  Product6/1 -> Sum3/1
  Product7/1 -> Sum3/2
  Sum3/1 -> Mux/4  "q3"
  psi/2/1 -> cos/1, sin/1
  tet/2/1 -> cos1/1, sin1/1
  gam/2/1 -> cos2/1, sin2/1
  Divide to normalize/1 -> Q/1
  Dot Product/1 -> Sqrt/1
  Sqrt/1 -> Divide to normalize/2

== system KIT_pr_UDR/Forces and Moments/Forces/Drag ==
  Alpha : Inport
  nv : Inport  Port=2
  q : Inport  Port=3
  Drag1 : Subsystem
  Gain : Gain  Gain=-1
  Product1 : Product
  Drag : Outport  VectorParamsAs1DForOutWhenUnconnected=off
  wires:
  Drag1/1(Drag) -> Product1/1
  nv/1 -> Product1/2
  q/1 -> Drag1/2(q)
  Alpha/1 -> Drag1/1(Alpha)
  Product1/1 -> Gain/1
  Gain/1 -> Drag/1

== system KIT_pr_UDR/Forces and Moments/Forces/Lift ==
  Alpha : Inport
  nv : Inport  Port=2
  q : Inport  Port=3
  Demux2 : Demux  Outputs=3
  "Lift " : Subsystem
  MATLAB Function1 : MATLAB Function  TreatAsAtomicUnit=on
  Product3 : Product
  Terminator4 : Terminator
  Vector Concatenate2 : Concatenate  NumInputs=3
  Lift : Outport  VectorParamsAs1DForOutWhenUnconnected=off
  wires:
  Demux2/3 -> Terminator4/1
  Vector Concatenate2/1 -> Product3/2
  Demux2/2 -> MATLAB Function1/2(Vy)
  MATLAB Function1/3(Lz) -> Vector Concatenate2/3
  MATLAB Function1/2(Ly) -> Vector Concatenate2/2
  "Lift "/1(Lift) -> Product3/1
  nv/1 -> Demux2/1
  MATLAB Function1/1(Lx) -> Vector Concatenate2/1
  Product3/1 -> Lift/1
  Demux2/1 -> MATLAB Function1/1(Vx)
  q/1 -> "Lift "/2(q)
  Alpha/1 -> "Lift "/1(alpha)

== system KIT_pr_UDR/Forces and Moments/Forces/Side Force ==
  q : Inport
  Beta : Inport  Port=2
  Constant2 : Constant  Value=0
  Mux : Mux  Inputs=3
  Product : Product  Inputs=3
  cz_beta : Constant  Value=-0.2469
  Side Force : Outport
  wires:
  q/1 -> Product/1
  Beta/1 -> Product/2
  Product/1 -> Mux/3
  Mux/1 -> Side Force/1
  Constant2/1 -> Mux/2, Mux/1
  cz_beta/1 -> Product/3

== system KIT_pr_UDR/Forces and Moments/Forces/Subsystem ==
  in : Inport
  Square : Math  Operator=square
  Square Root : Sqrt
  Square Root1 : Sqrt
  Sum of Elements : Sum  Inputs=+
  abs : Outport  VectorParamsAs1DForOutWhenUnconnected=off
  wires:
  in/1 -> Square/1
  Square/1 -> Sum of Elements/1
  Sum of Elements/1 -> Square Root1/1
  Square Root1/1 -> abs/1

== system KIT_pr_UDR/Forces and Moments/Forces/Subsystem1 ==
  in : Inport
  Square : Math  Operator=square
  Square Root : Sqrt
  Square Root1 : Sqrt
  Sum of Elements : Sum  Inputs=+
  abs : Outport  VectorParamsAs1DForOutWhenUnconnected=off
  wires:
  in/1 -> Square/1
  Square/1 -> Sum of Elements/1
  Sum of Elements/1 -> Square Root1/1
  Square Root1/1 -> abs/1

== system KIT_pr_UDR/Forces and Moments/Forces/Subsystem2 ==
  in : Inport
  Square : Math  Operator=square
  Square Root : Sqrt
  Square Root1 : Sqrt
  Sum of Elements : Sum  Inputs=+
  abs : Outport  VectorParamsAs1DForOutWhenUnconnected=off
  wires:
  in/1 -> Square/1
  Square/1 -> Sum of Elements/1
  Sum of Elements/1 -> Square Root1/1
  Square Root1/1 -> abs/1

== system KIT_pr_UDR/Forces and Moments/Forces/Subsystem3 ==
  in : Inport
  Square : Math  Operator=square
  Square Root : Sqrt
  Square Root1 : Sqrt
  Sum of Elements : Sum  Inputs=+
  abs : Outport  VectorParamsAs1DForOutWhenUnconnected=off
  wires:
  in/1 -> Square/1
  Square/1 -> Sum of Elements/1
  Sum of Elements/1 -> Square Root1/1
  Square Root1/1 -> abs/1

== system KIT_pr_UDR/Forces and Moments/Forces/Thrust ==
  Thrust(0..1) : Inport
  Vb : Inport  Port=2
  Constant : Constant  Value=0
  Formula Thrust : MATLAB Function  TreatAsAtomicUnit=on
  Subsystem : Subsystem
  Vector Concatenate : Concatenate  NumInputs=3
  Thrust : Outport  VectorParamsAs1DForOutWhenUnconnected=off
  wires:
  Subsystem/1(abs) -> Formula Thrust/2(V)
  Vb/1 -> Subsystem/1(in)
  Thrust(0..1)/1 -> Formula Thrust/1(x)
  Vector Concatenate/1 -> Thrust/1
  Formula Thrust/1(T) -> Vector Concatenate/1
  Constant/1 -> Vector Concatenate/2, Vector Concatenate/3

== system KIT_pr_UDR/Forces and Moments/Forces/Weight ==
  Mass : Inport
  Matrix E->B : Inport  Port=2
  Constant2 : Constant  Value=[0 -9.8 0]
  Product2 : Product
  Weight1 : Product  Multiplication=Matrix(*)
  Weight : Outport  VectorParamsAs1DForOutWhenUnconnected=off
  wires:
  Constant2/1 -> Product2/1
  Mass/1 -> Product2/2
  Weight1/1 -> Weight/1
  Matrix E->B/1 -> Weight1/1
  Product2/1 -> Weight1/2

== system KIT_pr_UDR/Forces and Moments/Moments/LiftMoment ==
  Alpha(Rad) : Inport
  q : Inport  Port=2
  ang_vel : Inport  Port=3
  Angle Conversion : aerolibconvert2/Angle Conversion  IU=rad  OU=deg
  Constant : Constant  Value=0
  Subsystem2 : Subsystem
  Vector Concatenate : Concatenate  NumInputs=3
  M : Outport  VectorParamsAs1DForOutWhenUnconnected=off
  wires:
  q/1 -> Subsystem2/2(q)
  Angle Conversion/1 -> Subsystem2/1(Alpha)
  Alpha(Rad)/1 -> Angle Conversion/1
  Subsystem2/1(Mz) -> Vector Concatenate/3
  Vector Concatenate/1 -> M/1
  Constant/1 -> Vector Concatenate/2, Vector Concatenate/1
  ang_vel/1 -> Subsystem2/3(ang_vel)

== system KIT_pr_UDR/Forces and Moments/Moments/RollMoment ==
  ang_vel : Inport
  q : Inport  Port=2
  Constant : Constant  Value=0
  Divide : Product  Inputs=**
  Product1 : Product
  Selector : Selector  InputPortWidth=3  IndexOptions=Index vector (dialog)  Indices=[1]  OutputSizes=1
  Vector Concatenate : Concatenate  NumInputs=3
  mx_wx : Constant  Value=-0.3097
  M : Outport  VectorParamsAs1DForOutWhenUnconnected=off
  wires:
  Constant/1 -> Vector Concatenate/3, Vector Concatenate/2
  Vector Concatenate/1 -> M/1
  Selector/1 -> Divide/1
  ang_vel/1 -> Selector/1
  mx_wx/1 -> Divide/2
  q/1 -> Product1/2
  Divide/1 -> Product1/1
  Product1/1 -> Vector Concatenate/1

== system KIT_pr_UDR/Forces and Moments/Moments/SideForceMoment ==
  Beta : Inport
  ang_vel : Inport  Port=2
  q : Inport  Port=3
  Constant : Constant  Value=0
  Divide : Product  Inputs=**
  Product : Product
  Product1 : Product
  Selector : Selector  InputPortWidth=3  IndexOptions=Index vector (dialog)  Indices=[2]  OutputSizes=1
  Sum : Sum
  Vector Concatenate : Concatenate  NumInputs=3
  my_beta : Constant  Value=-0.1858
  my_wy2 : Constant  Value=-0.073
  M : Outport  VectorParamsAs1DForOutWhenUnconnected=off
  wires:
  Constant/1 -> Vector Concatenate/3, Vector Concatenate/1
  Vector Concatenate/1 -> M/1
  Beta/1 -> Product/1
  my_beta/1 -> Product/2
  Selector/1 -> Divide/1
  ang_vel/1 -> Selector/1
  q/1 -> Product1/2
  Product/1 -> Sum/2
  Sum/1 -> Product1/1
  Product1/1 -> Vector Concatenate/2
  Divide/1 -> Sum/1
  my_wy2/1 -> Divide/2

== system KIT_pr_UDR/Forces and Moments/alpha, beta, V direction vector/Subsystem ==
  in : Inport
  Sqrt : Sqrt
  Square : Math  Operator=square
  Sum of Elements : Sum  Inputs=+
  abs : Outport  VectorParamsAs1DForOutWhenUnconnected=off
  wires:
  in/1 -> Square/1
  Square/1 -> Sum of Elements/1
  Sum of Elements/1 -> Sqrt/1
  Sqrt/1 -> abs/1

== system KIT_pr_UDR/Forces and Moments/alpha, beta, V direction vector/Subsystem4 ==
  V : Inport
  Demux1 : Demux  Outputs=3
      settings: DisplayOption=none
  Terminator : Terminator
  y : Outport  VectorParamsAs1DForOutWhenUnconnected=off
  x : Outport  Port=2  VectorParamsAs1DForOutWhenUnconnected=off
  wires:
  Demux1/1 -> x/1
  Demux1/2 -> y/1
  V/1 -> Demux1/1
  Demux1/3 -> Terminator/1

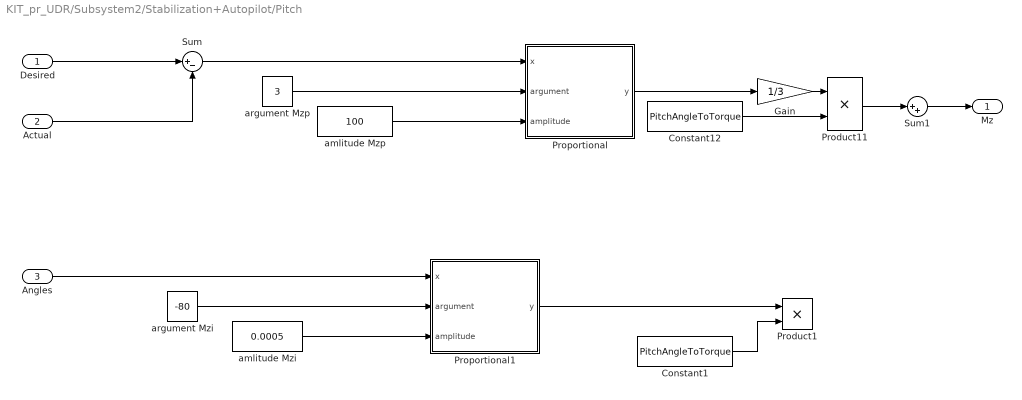
== system KIT_pr_UDR/Subsystem2/Stabilization+Autopilot/Pitch ==
  Desired : Inport
  Actual : Inport  Port=2
  Angles : Inport  Port=3
  Constant1 : Constant  Value=PitchAngleToTorque
  Constant12 : Constant  Value=PitchAngleToTorque
  Gain : Gain  Gain=1/3
  Product1 : Product
  Product11 : Product
  Proportional : MATLAB Function  TreatAsAtomicUnit=on
  Proportional1 : MATLAB Function  TreatAsAtomicUnit=on
  Sum : Sum  Inputs=|+-
  Sum1 : Sum  Inputs=|++
  amlitude Mzi : Constant  Value=0.0005
  amlitude Mzp : Constant  Value=100
  argument Mzi : Constant  Value=-80
  argument Mzp : Constant  Value=3
  Mz : Outport
  wires:
  Desired/1 -> Sum/1
  Sum/1 -> Proportional/1(x)
  Actual/1 -> Sum/2
  argument Mzp/1 -> Proportional/2(argument)
  amlitude Mzp/1 -> Proportional/3(amplitude)
  Constant12/1 -> Product11/2
  Gain/1 -> Product11/1
  Product11/1 -> Sum1/1
  Proportional/1(y) -> Gain/1
  amlitude Mzi/1 -> Proportional1/3(amplitude)
  Constant1/1 -> Product1/2
  argument Mzi/1 -> Proportional1/2(argument)
  Proportional1/1(y) -> Product1/1
  Angles/1 -> Proportional1/1(x)
  Sum1/1 -> Mz/1

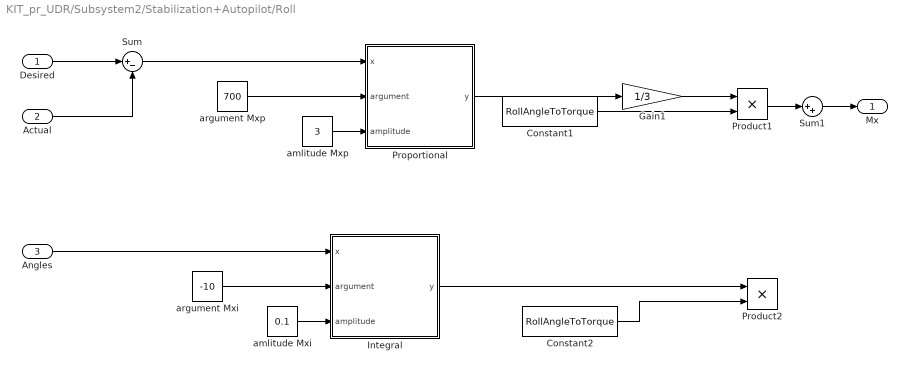
== system KIT_pr_UDR/Subsystem2/Stabilization+Autopilot/Roll ==
  Desired : Inport
  Actual : Inport  Port=2
  Angles : Inport  Port=3
  Constant1 : Constant  Value=RollAngleToTorque
  Constant2 : Constant  Value=RollAngleToTorque
  Gain1 : Gain  Gain=1/3
  Integral : MATLAB Function  TreatAsAtomicUnit=on
  Product1 : Product
  Product2 : Product
  Proportional : MATLAB Function  TreatAsAtomicUnit=on
  Sum : Sum  Inputs=|+-
  Sum1 : Sum  Inputs=|++
  amlitude Mxi : Constant  Value=0.1
  amlitude Mxp : Constant  Value=3
  argument Mxi : Constant  Value=-10
  argument Mxp : Constant  Value=700
  Mx : Outport
  wires:
  Desired/1 -> Sum/1
  Actual/1 -> Sum/2
  Sum/1 -> Proportional/1(x)
  amlitude Mxp/1 -> Proportional/3(amplitude)
  Constant1/1 -> Product1/2
  Proportional/1(y) -> Gain1/1
  Gain1/1 -> Product1/1
  Product1/1 -> Sum1/1
  argument Mxp/1 -> Proportional/2(argument)
  Sum1/1 -> Mx/1
  Integral/1(y) -> Product2/1
  argument Mxi/1 -> Integral/2(argument)
  amlitude Mxi/1 -> Integral/3(amplitude)
  Constant2/1 -> Product2/2
  Angles/1 -> Integral/1(x)

== system KIT_pr_UDR/Subsystem2/Stabilization+Autopilot/Subsystem ==
  V : Inport
  Demux1 : Demux  Outputs=3
  Product : Product  RndMeth=Zero
  Product1 : Product  RndMeth=Zero
  Product2 : Product  RndMeth=Zero
  Sum : Sum  Inputs=+++
  abs : Outport  VectorParamsAs1DForOutWhenUnconnected=off
  wires:
  Demux1/1 -> Product/2, Product/1
  Demux1/2 -> Product1/1, Product1/2
  Product1/1 -> Sum/2
  Product2/1 -> Sum/3
  V/1 -> Demux1/1
  Demux1/3 -> Product2/2, Product2/1
  Product/1 -> Sum/1
  Sum/1 -> abs/1

== system KIT_pr_UDR/Subsystem2/Stabilization+Autopilot/Yaw ==
  Acceleration : Inport
  Constant1 : Constant  Value=YawAngleToTorque
  Desired acceleration : Constant  Value=0
  Gain1 : Gain  Gain=1/3
  Product1 : Product
  Proportional1 : MATLAB Function  TreatAsAtomicUnit=on
  Sum2 : Sum  Inputs=|+-
  amlitude Mzp1 : Constant  Value=3
  argument Mzp2 : Constant
  Mz : Outport
  wires:
  Product1/1 -> Mz/1
  Gain1/1 -> Product1/1
  amlitude Mzp1/1 -> Proportional1/3(amplitude)
  argument Mzp2/1 -> Proportional1/2(argument)
  Sum2/1 -> Proportional1/1(x)
  Constant1/1 -> Product1/2
  Acceleration/1 -> Sum2/2
  Desired acceleration/1 -> Sum2/1
  Proportional1/1(y) -> Gain1/1

== system KIT_pr_UDR/Subsystem2/Stabilization+Autopilot1/Subsystem ==
  in : Inport
  Square : Math  Operator=square
  Sum of Elements : Sum  Inputs=+
  abs : Outport  VectorParamsAs1DForOutWhenUnconnected=off
  wires:
  in/1 -> Square/1
  Square/1 -> Sum of Elements/1
  Sum of Elements/1 -> abs/1

== system KIT_pr_UDR/Subsystem2/Thrust/Subsystem ==
  in : Inport
  Sqrt : Sqrt
  Sqrt1 : Sqrt
  Square : Math  Operator=square
  Sum of Elements : Sum  Inputs=+
  abs : Outport  VectorParamsAs1DForOutWhenUnconnected=off
  wires:
  in/1 -> Square/1
  Square/1 -> Sum of Elements/1
  Sum of Elements/1 -> Sqrt1/1
  Sqrt1/1 -> abs/1

== system KIT_pr_UDR/Forces and Moments/Forces/Drag/Drag1 ==
  Alpha : Inport
  q : Inport  Port=2
  Constant : Constant  Value=Cx_alpha
  Constant1 : Constant  Value=square
  Polynomial Evaluation : dsppolyfun/Polynomial Evaluation  useConstCoeffs=off  constCoeffs=[5 4 3 2 1]
  Product : Product  Inputs=3
  Drag : Outport  VectorParamsAs1DForOutWhenUnconnected=off
  wires:
  Polynomial Evaluation/1 -> Product/2
  Product/1 -> Drag/1
  Alpha/1 -> Polynomial Evaluation/1
  Constant/1 -> Polynomial Evaluation/2
  q/1 -> Product/1
  Constant1/1 -> Product/3

== system KIT_pr_UDR/Forces and Moments/Forces/Lift/Lift  ==
  alpha : Inport
  q : Inport  Port=2
  Constant : Constant  Value=Cy_alpha
  Polynomial Evaluation : dsppolyfun/Polynomial Evaluation  useConstCoeffs=off  constCoeffs=[5 4 3 2 1]
  Product : Product  Inputs=3
  Wng_square : Constant  Value=square
  Lift : Outport  VectorParamsAs1DForOutWhenUnconnected=off
  wires:
  Product/1 -> Lift/1
  Polynomial Evaluation/1 -> Product/2
  alpha/1 -> Polynomial Evaluation/1
  Constant/1 -> Polynomial Evaluation/2
  q/1 -> Product/1
  Wng_square/1 -> Product/3

== system KIT_pr_UDR/Forces and Moments/Forces/Thrust/Subsystem ==
  in : Inport
  Square : Math  Operator=square
  Sum of Elements : Sum  Inputs=+
  abs : Outport  VectorParamsAs1DForOutWhenUnconnected=off
  wires:
  in/1 -> Square/1
  Square/1 -> Sum of Elements/1
  Sum of Elements/1 -> abs/1

== system KIT_pr_UDR/Forces and Moments/Moments/LiftMoment/Subsystem2 ==
  Alpha : Inport
  q : Inport  Port=2
  ang_vel : Inport  Port=3
  Constant : Constant  Value=mz_alpha
  Constant2 : Constant  Value=square
  Divide : Product  Inputs=**
  Polynomial Evaluation : dsppolyfun/Polynomial Evaluation  useConstCoeffs=off  constCoeffs=[5 4 3 2 1]
  Product : Product  Inputs=3
  Selector : Selector  InputPortWidth=3  IndexOptions=Index vector (dialog)  Indices=[3]  OutputSizes=1
  Sum : Sum
  mz_wz : Constant  Value=-0.0493
  Mz : Outport  VectorParamsAs1DForOutWhenUnconnected=off
  wires:
  Constant/1 -> Polynomial Evaluation/2
  Alpha/1 -> Polynomial Evaluation/1
  Product/1 -> Mz/1
  Polynomial Evaluation/1 -> Sum/2
  Sum/1 -> Product/1
  Constant2/1 -> Product/3
  ang_vel/1 -> Selector/1
  Selector/1 -> Divide/1
  mz_wz/1 -> Divide/2
  Divide/1 -> Sum/1
  q/1 -> Product/2

== matlab function KIT_pr_UDR/Forces and Moments/Forces/Lift/MATLAB Function1 ==
  data: Vx input; Lx output; Vy input; Ly output; Lz output
function [Lx,Ly,Lz]= fcn(Vx,Vy)
Lz=0;
if (Vx*Vx+Vy*Vy==0)
    Lx=0;
    Ly=1;
else 
    Lx=-Vy/sqrt(Vx*Vx+Vy*Vy);
    Ly=Vx/sqrt(Vx*Vx+Vy*Vy);
end
end

== matlab function KIT_pr_UDR/Subsystem2/Thrust/MATLAB Function ==
  data: x input; y output; argument input; amplitude input
function y = fcn(x,argument,amplitude)

y = amplitude*atan(x*argument)/(pi/2)
if y<0
    y=0;
end

== matlab function KIT_pr_UDR/Subsystem2/Stabilization+Autopilot1/MATLAB Function1 ==
  data: alpha input; mz output; delta input
function mz = fcn(alpha,delta)
%function from solidworks
mz = (-0.0001 * alpha^2  + 0.054) * delta * 2 / (625 * 1.225);

== matlab function KIT_pr_UDR/Calculations1/Bazhenov fun ==
  data: roll input; pitch input; yaw input; EtoB output
function EtoB = A(roll,pitch,yaw)
EtoB = zeros(3,3);
EtoB(1,1)=cos(pitch)*cos(yaw)
EtoB(1,2)=sin(pitch)
EtoB(1,3)=sin(yaw)*cos(pitch)
EtoB(2,1)=-cos(yaw)*sin(pitch)*cos(roll)-sin(yaw)*sin(roll)
EtoB(2,2)=cos(pitch)*cos(roll)
EtoB(2,3)=-sin(yaw)*sin(pitch)*cos(roll)+cos(yaw)*sin(roll)
EtoB(3,1)=cos(yaw)*sin(pitch)*sin(roll)-sin(yaw)*cos(roll)
EtoB(3,2)=-cos(pitch)*sin(roll)
EtoB(3,3)=sin(yaw)*sin(pitch)*sin(roll)+cos(roll)*cos(yaw)
end

== matlab function KIT_pr_UDR/Subsystem2/Stabilization+Autopilot/Yaw/Proportional1 ==
  data: x input; y output; argument input; amplitude input
function y = fcn(x,argument,amplitude)

y = amplitude*atan(x*argument)/(pi/2)
end

== matlab function KIT_pr_UDR/Subsystem2/Stabilization+Autopilot1/MATLAB Function2 ==
  data: beta input; my output; delta input
function my = fcn(beta,delta)
%function from xfoil calc
my = (6.638130252100894*(10^-5)* beta^2  + 0.0022921481092436874 * beta - 0.06407503676470584) * delta * 0.021 * 0.77;

== matlab function KIT_pr_UDR/Subsystem2/Stabilization+Autopilot1/MATLAB Function ==
  data: alpha input; mx output; delta input
function mx = fcn(alpha,delta)
%function from xfoil, delta, arm, two ailerons,square
mx = (-1.6182*(10^-4) * alpha^2 - 0.0023 * alpha + 0.0695) * delta * 0.691 * 2 * 0.0446;

== matlab function KIT_pr_UDR/Subsystem2/Stabilization+Autopilot/Pitch/Proportional ==
  data: x input; y output; argument input; amplitude input
function y = fcn(x,argument,amplitude)

y = amplitude*atan(x*argument)/(pi/2)
end

== matlab function KIT_pr_UDR/Subsystem2/Stabilization+Autopilot/Roll/Integral ==
  data: x input; y output; argument input; amplitude input
function y = fcn(x,argument,amplitude)

y = amplitude*atan(x*argument)/(pi/2)
end

== matlab function KIT_pr_UDR/Subsystem2/Stabilization+Autopilot/Pitch/Proportional1 ==
  data: x input; y output; argument input; amplitude input
function y = fcn(x,argument,amplitude)

y = amplitude*atan(x*argument)/(pi/2)
end

== matlab function KIT_pr_UDR/Subsystem2/Stabilization+Autopilot/Roll/Proportional ==
  data: x input; y output; argument input; amplitude input
function y = fcn(x,argument,amplitude)

y = amplitude*atan(x*argument)/(pi/2)
end

== matlab function KIT_pr_UDR/Forces and Moments/Forces/Thrust/Formula Thrust ==
  data: x input; T output; V input
function T = thrust(x,V)
if (x<0) x=0;
end
T=(39.2-0.98*V)*x;
if (T<0) T = 0; 
end
end
